simulink model "part1"  (R2025a)
settings: Solver=FixedStepAuto  StartTime=0.0  StopTime=t_end  FixedStep=dt  RelTol=1e-3
values from neighbouring files (symbols this model uses):
  alpha = wind_coeff(:,1)*pi/180    [windCoefficients.m]
  C_pitch = wind_coeff(:,6)    [windCoefficients.m]
  C_roll = wind_coeff(:,5)    [windCoefficients.m]
  C_yaw = wind_coeff(:,7)    [windCoefficients.m]
  Cx = wind_coeff(:,2)    [windCoefficients.m]
  Cy = wind_coeff(:,3)    [windCoefficients.m]
  Cz = wind_coeff(:,4)    [windCoefficients.m]
  Kd = diag([9.3e5 7e5 4e6])    [init.m]
  Ki = diag([8.5e3 7.5e3 3.5e4])    [init.m]
  Kp = diag([7.8e5   9.8e5   1.5e8])    [init.m]    (also in init_pid.m = M*Omega_n^2)
  mu = 0.001    [SimulationParam.m]
  U_bar = 10    [SimulationParam.m]
  Vc = -0.2    [SimulationParam.m]
  vessel = computeManeuveringModel(vessel, omega_p, plotFlag)    [init_pid.m]
undefined symbols (not defined in the file or in its folder): currentMode, DiscIntNeverNeededParam, Hoerner, thrusters, windFlag
libraries: marine_gnc x1, marine_hydro x1, simulink x1
settings Model: Creator=jonbjor  LastModifiedBy=evenf
settings SolverCC: AlgebraicLoopSolver=TrustRegion
settings DataIOCC: ReturnWorkspaceOutputs=off
settings DebuggingCC: UnconnectedInputMsg=warning  UnconnectedOutputMsg=warning  UnconnectedLineMsg=warning  ArithmeticOperatorsInVariantConditions=warning
settings ModelReferenceCC: EnableRefExpFcnMdlSchedulingChecks=on
settings SFSimCC: SimUseLocalCustomCode=off  CustomCodeUndefinedFunction=UseInterfaceOnly
settings RTWCC: RTWUseLocalCustomCode=off  GPUComputeCapability=3.5  DLArmComputeVersion=19.05

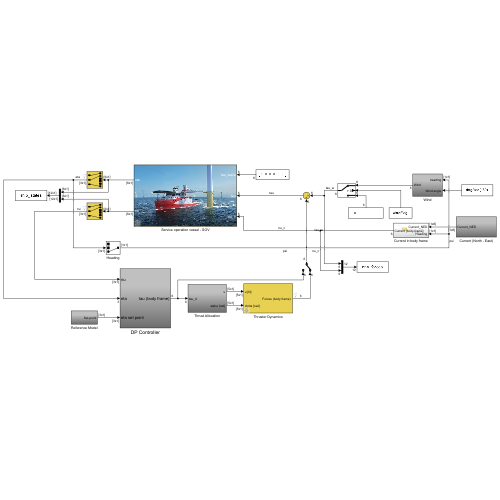
[thumbnail: Simulink's stored preview of the top-level diagram]
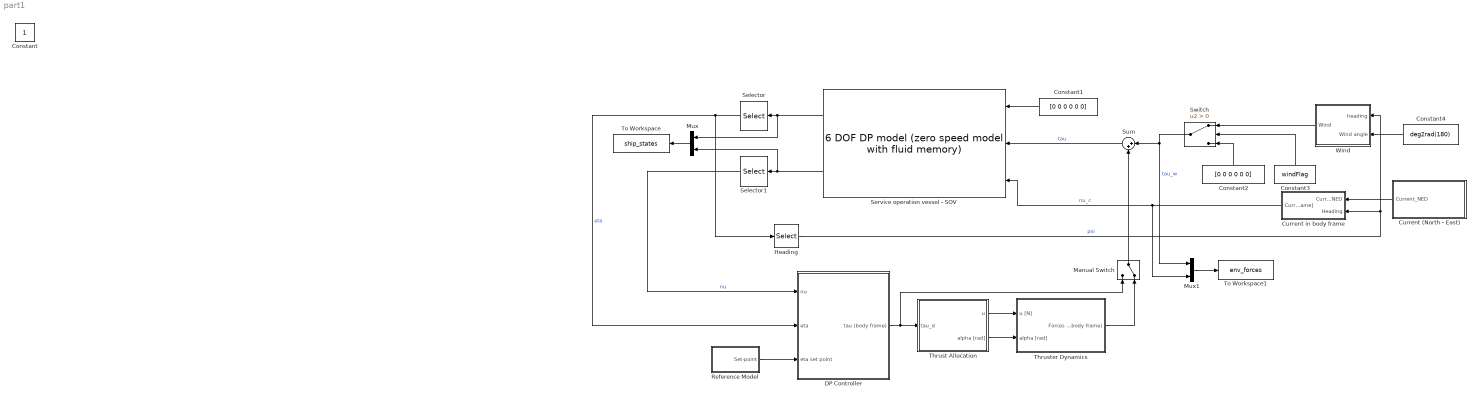
== system part1 ==
  Constant1 : Constant  Value=[0 0 0 0 0 0]
  Constant2 : Constant  Value=[0 0 0 0 0 0]
  Constant3 : Constant  Value=windFlag
  Constant4 : Constant  Value=deg2rad(180)
  Current (North - East) : Subsystem
  Current in body frame : Subsystem
  DP Controller : Subsystem
  Heading : Selector  InputPortWidth=3  IndexOptions=Index vector (dialog)  Indices=[3]  OutputSizes=1
  Manual Switch : ManualSwitch  CurrentSetting=0
  Mux : Mux  Inputs=2
  Mux1 : Mux  Inputs=2
  Reference Model : Subsystem
  Selector : Selector  InputPortWidth=6  IndexOptions=Index vector (dialog)  Indices=[1 2 6]  OutputSizes=1
  Selector1 : Selector  InputPortWidth=6  IndexOptions=Index vector (dialog)  Indices=[1 2 6]  OutputSizes=1
  Service operation vessel - SOV : marine_hydro/Hydro Library/6 DOF DP model  (zero speed model with fluid memory)  ABC=vesselABC  rho=1025  Axc=0.9*vessel.main.T*vessel.main.B  Ayc=0.9*vessel.main.T*vessel.main.Lpp  CX=1  CY_2D=Hoerner(vessel.main.B,vessel.main.T)  Bv=vessel.Bv  mask(6 DOF zero speed model){}
      link override "Integrator1 ": InitialCondition=nu0
      link override Integrator2: InitialCondition=eta0
      settings: SourceProductName=MSS Hydro
      mask Display:
      | image('SOV.jpg');
      | color('white'); port_label('output', 1, 'eta')
      | color('white'); port_label('output', 2, 'nu')
      | color('white'); port_label('input', 1, 'tau_wave')
      | color('white'); port_label('input', 2, 'tau')
      | color('white'); port_label('input', 3, 'nu_c')
  Sum : Sum  Inputs=|++
  Switch : Switch  Criteria=u2 > Threshold  SaturateOnIntegerOverflow=off  InputSameDT=off
  Thrust Allocation : Subsystem
  Thruster Dynamics : Subsystem  mask{thrusterfault=off}
      mask prompts: thrusterfault "Fault on thruster #2 and #4?"
  To Workspace : ToWorkspace  VariableName=ship_states  SampleTime=-1
  To Workspace1 : ToWorkspace  VariableName=env_forces  SampleTime=-1
      settings: Save2DSignal=2-D array (concatenate along first dimension)
  Wind : Subsystem
  Constant : Constant  IOType=siggen
  wires:
  Service operation vessel - SOV/1 -> Mux/1, Selector/1
  Service operation vessel - SOV/2 -> Mux/2, Selector1/1
  Selector/1 -> Heading/1, DP Controller/2(eta)  "eta"
  Selector1/1 -> DP Controller/1(nu)  "nu"
  Thrust Allocation/1(u) -> Thruster Dynamics/1(u [N])
  Thrust Allocation/2(alpha [rad]) -> Thruster Dynamics/2(alpha [rad])
  DP Controller/1(tau (body frame)) -> Thrust Allocation/1(tau_d), Manual Switch/1
  Sum/1 -> Service operation vessel - SOV/2  "tau"
  Current (North - East)/1(Current_NED) -> Current in body frame/1(Current_NED)
  Heading/1 -> Current in body frame/2(Heading), Wind/1(heading)  "psi"
  Current in body frame/1(Current [body-frame]) -> Service operation vessel - SOV/3, Mux1/2  "nu_c"
  Switch/1 -> Sum/1, Mux1/1  "tau_w"
  Manual Switch/1 -> Sum/2
  Thruster Dynamics/1("Forces (body frame) ") -> Manual Switch/2
  Reference Model/1(Set-point) -> DP Controller/3(eta set point)
  Mux/1 -> To Workspace/1
  Mux1/1 -> To Workspace1/1
  Constant3/1 -> Switch/2
  Constant2/1 -> Switch/3
  Wind/1(Wind) -> Switch/1
  Constant1/1 -> Service operation vessel - SOV/1
  Constant4/1 -> Wind/2(Wind angle)

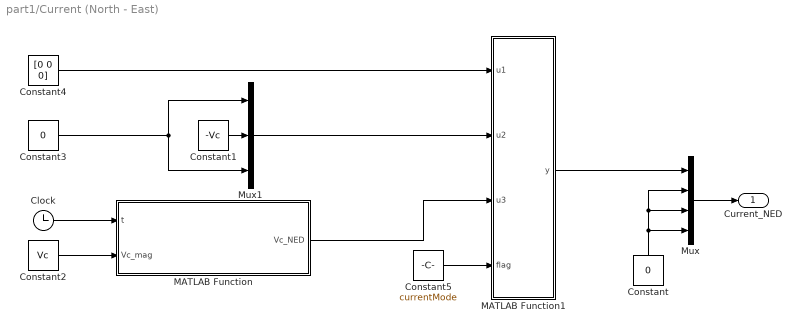
== system part1/Current (North - East) ==
  Clock : Clock
  Constant : Constant  Value=0
  Constant1 : Constant  Value=-Vc
  Constant2 : Constant  Value=Vc
  Constant3 : Constant  Value=0
  Constant4 : Constant  Value=[0 0 0]
  Constant5 : Constant  Value=currentMode
  MATLAB Function : MATLAB Function  TreatAsAtomicUnit=on
  MATLAB Function1 : MATLAB Function  TreatAsAtomicUnit=on
  Mux : Mux
  Mux1 : Mux  Inputs=3
  Current_NED : Outport  VectorParamsAs1DForOutWhenUnconnected=off
  wires:
  Constant1/1 -> Mux1/2
  Constant3/1 -> Mux1/1, Mux1/3
  Clock/1 -> MATLAB Function/1(t)
  Constant2/1 -> MATLAB Function/2(Vc_mag)
  Mux/1 -> Current_NED/1
  Constant/1 -> Mux/2, Mux/3, Mux/4
  Mux1/1 -> MATLAB Function1/2(u2)
  MATLAB Function/1(Vc_NED) -> MATLAB Function1/3(u3)
  Constant4/1 -> MATLAB Function1/1(u1)
  Constant5/1 -> MATLAB Function1/4(flag)
  MATLAB Function1/1(y) -> Mux/1

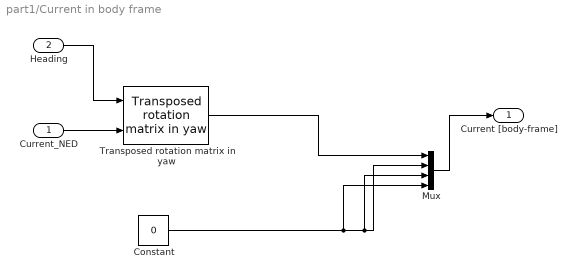
== system part1/Current in body frame ==
  Current_NED : Inport
  Heading : Inport  Port=2
  Constant : Constant  Value=0
  Mux : Mux
  Transposed rotation matrix in yaw : marine_gnc/Models/ Kinematics/Transposed rotation  matrix in yaw
      settings: SourceProductName=MSS GNC
  Current [body-frame] : Outport
  wires:
  Current_NED/1 -> Transposed rotation matrix in yaw/2
  Transposed rotation matrix in yaw/1 -> Mux/1
  Heading/1 -> Transposed rotation matrix in yaw/1
  Mux/1 -> Current [body-frame]/1
  Constant/1 -> Mux/4, Mux/3, Mux/2

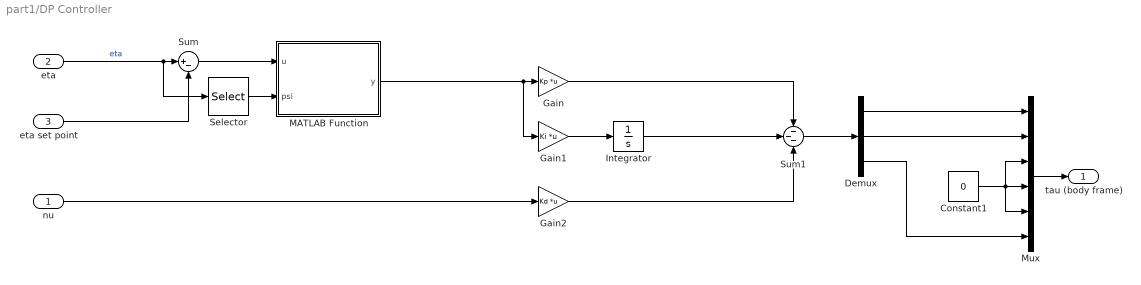
== system part1/DP Controller ==
  nu : Inport
  eta : Inport  Port=2
  eta set point : Inport  Port=3
  Constant1 : Constant  Value=0
  Demux : Demux  Outputs=3
  Gain : Gain  Gain=Kp  Multiplication=Matrix(K*u)
  Gain1 : Gain  Gain=Ki  Multiplication=Matrix(K*u)
  Gain2 : Gain  Gain=Kd  Multiplication=Matrix(K*u)
  Integrator : Integrator
  MATLAB Function : MATLAB Function  TreatAsAtomicUnit=on
  Mux : Mux  Inputs=6
  Selector : Selector  InputPortWidth=3  IndexOptions=Index vector (dialog)  Indices=[3]  OutputSizes=1
  Sum : Sum  Inputs=|+-
  Sum1 : Sum  Inputs=---
  tau (body frame) : Outport  VectorParamsAs1DForOutWhenUnconnected=off
  wires:
  Mux/1 -> tau (body frame)/1
  Constant1/1 -> Mux/5, Mux/3, Mux/4
  eta/1 -> Selector/1, Sum/1  "eta"
  eta set point/1 -> Sum/2
  Selector/1 -> MATLAB Function/2(psi)
  Sum/1 -> MATLAB Function/1(u)
  MATLAB Function/1(y) -> Gain1/1, Gain/1
  Gain1/1 -> Integrator/1
  Integrator/1 -> Sum1/2
  Gain/1 -> Sum1/1
  Sum1/1 -> Demux/1
  Demux/1 -> Mux/1
  Demux/3 -> Mux/6
  Demux/2 -> Mux/2
  nu/1 -> Gain2/1
  Gain2/1 -> Sum1/3

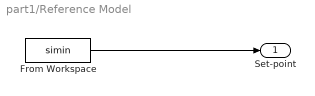
== system part1/Reference Model ==
  From Workspace : FromWorkspace  VariableName=simin
  Set-point : Outport  VectorParamsAs1DForOutWhenUnconnected=off
  wires:
  From Workspace/1 -> Set-point/1

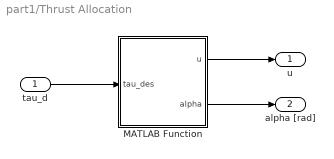
== system part1/Thrust Allocation ==
  tau_d : Inport
  MATLAB Function : MATLAB Function  TreatAsAtomicUnit=on
  u : Outport  VectorParamsAs1DForOutWhenUnconnected=off
  alpha [rad] : Outport  Port=2  VectorParamsAs1DForOutWhenUnconnected=off
  wires:
  MATLAB Function/1(u) -> u/1
  MATLAB Function/2(alpha) -> alpha [rad]/1
  tau_d/1 -> MATLAB Function/1(tau_des)

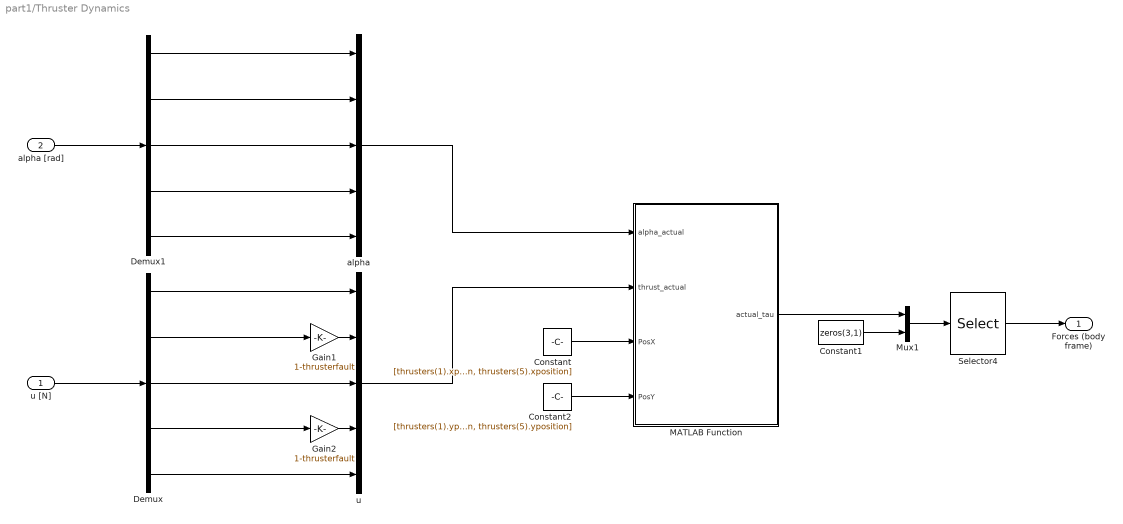
== system part1/Thruster Dynamics ==
  u [N] : Inport
  alpha [rad] : Inport  Port=2
  Constant : Constant  Value=[thrusters(1).xposition, thrusters(2).xposition, thrusters(3).xposition, thrusters(4).xposition, thrusters(5).xposition]
  Constant1 : Constant  Value=zeros(3,1)
  Constant2 : Constant  Value=[thrusters(1).yposition, thrusters(2).yposition, thrusters(3).yposition, thrusters(4).yposition, thrusters(5).yposition]
  Demux : Demux  Outputs=5
  Demux1 : Demux  Outputs=5
  Gain1 : Gain  Gain=1-thrusterfault
  Gain2 : Gain  Gain=1-thrusterfault
  MATLAB Function : MATLAB Function  TreatAsAtomicUnit=on
  Mux1 : Mux  Inputs=2
  Selector4 : Selector  InputPortWidth=6  IndexOptions=Index vector (dialog)  Indices=[1 2 4 5 6 3]  OutputSizes=1
  alpha : Mux  Inputs=5
  u : Mux  Inputs=5
  "Forces (body frame) " : Outport  VectorParamsAs1DForOutWhenUnconnected=off
  wires:
  Mux1/1 -> Selector4/1
  Constant1/1 -> Mux1/2
  Selector4/1 -> "Forces (body frame) "/1
  Gain1/1 -> u/2
  u [N]/1 -> Demux/1
  alpha [rad]/1 -> Demux1/1
  Constant/1 -> MATLAB Function/3(PosX)
  Constant2/1 -> MATLAB Function/4(PosY)
  u/1 -> MATLAB Function/2(thrust_actual)
  alpha/1 -> MATLAB Function/1(alpha_actual)
  MATLAB Function/1(actual_tau) -> Mux1/1
  Demux1/1 -> alpha/1
  Gain2/1 -> u/4
  Demux/1 -> u/1
  Demux/2 -> Gain1/1
  Demux/3 -> u/3
  Demux/4 -> Gain2/1
  Demux/5 -> u/5
  Demux1/2 -> alpha/2
  Demux1/4 -> alpha/4
  Demux1/5 -> alpha/5
  Demux1/3 -> alpha/3

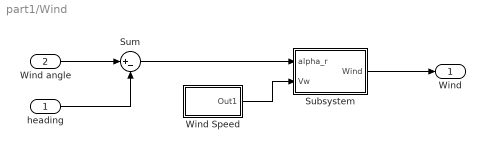
== system part1/Wind ==
  heading : Inport
  Wind angle : Inport  Port=2
  Subsystem : Subsystem
  Sum : Sum  Inputs=|+-
  Wind Speed : Subsystem
  Wind : Outport  VectorParamsAs1DForOutWhenUnconnected=off
  wires:
  Subsystem/1(Wind) -> Wind/1
  Wind Speed/1(Out1) -> Subsystem/2(Vw)
  Wind angle/1 -> Sum/1
  heading/1 -> Sum/2
  Sum/1 -> Subsystem/1(alpha_r)

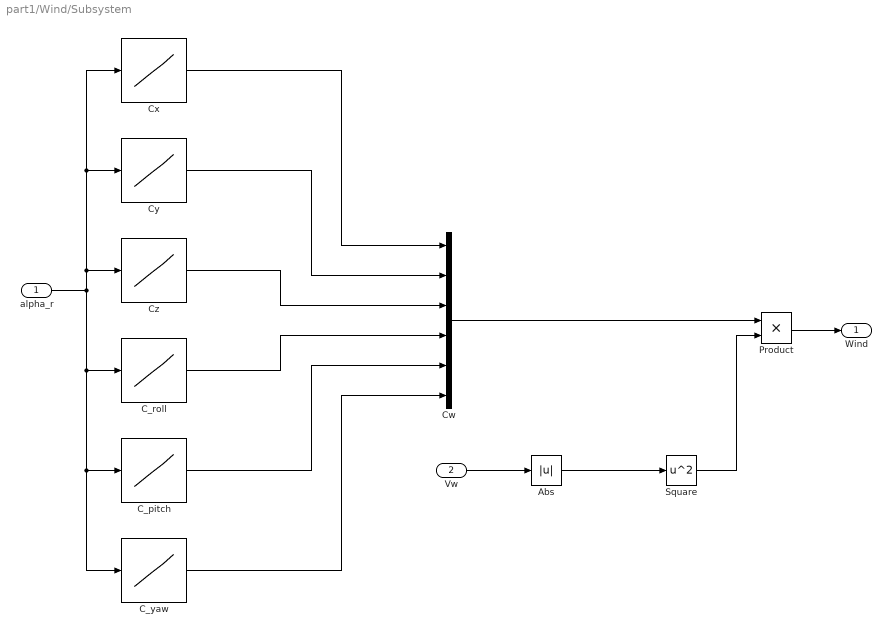
== system part1/Wind/Subsystem ==
  alpha_r : Inport
  Vw : Inport  Port=2
  Abs : Abs  SaturateOnIntegerOverflow=off
  C_pitch : Lookup_n-D  NumberOfTableDimensions=1  BreakpointsForDimension1=alpha  Table=C_pitch  InternalRulePriority=Speed  RndMeth=Simplest
  C_roll : Lookup_n-D  NumberOfTableDimensions=1  BreakpointsForDimension1=alpha  Table=C_roll  InternalRulePriority=Speed  RndMeth=Simplest
  C_yaw : Lookup_n-D  NumberOfTableDimensions=1  BreakpointsForDimension1=alpha  Table=C_yaw  InternalRulePriority=Speed  RndMeth=Simplest
  Cw : Mux  Inputs=6
  Cx : Lookup_n-D  NumberOfTableDimensions=1  BreakpointsForDimension1=alpha  Table=Cx  InternalRulePriority=Speed  RndMeth=Simplest
  Cy : Lookup_n-D  NumberOfTableDimensions=1  BreakpointsForDimension1=alpha  Table=Cy  InternalRulePriority=Speed  RndMeth=Simplest
  Cz : Lookup_n-D  NumberOfTableDimensions=1  BreakpointsForDimension1=alpha  Table=Cz  InternalRulePriority=Speed  RndMeth=Simplest
  Product : Product
  Square : Math  Operator=square
  Wind : Outport  VectorParamsAs1DForOutWhenUnconnected=off
  wires:
  Vw/1 -> Abs/1
  Cy/1 -> Cw/2
  C_roll/1 -> Cw/4
  Cw/1 -> Product/1
  C_pitch/1 -> Cw/5
  Square/1 -> Product/2
  alpha_r/1 -> C_yaw/1, C_pitch/1, C_roll/1, Cx/1, Cy/1, Cz/1
  Cz/1 -> Cw/3
  C_yaw/1 -> Cw/6
  Cx/1 -> Cw/1
  Abs/1 -> Square/1
  Product/1 -> Wind/1

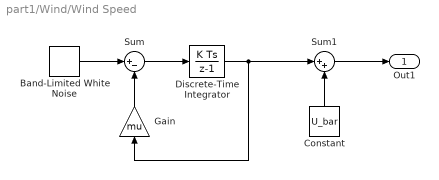
== system part1/Wind/Wind Speed ==
  Band-Limited White Noise : simulink/Sources/Band-Limited White Noise  Cov=power_w_c  Ts=0.1  seed=[23341]
  Constant : Constant  Value=U_bar
  Discrete-Time Integrator : DiscreteIntegrator  SampleTime=-1  ICPrevOutput=DiscIntNeverNeededParam  ICPrevScaledInput=DiscIntNeverNeededParam
  Gain : Gain  Gain=mu
  Sum : Sum  Inputs=|+-
  Sum1 : Sum  Inputs=|++
  Out1 : Outport
  wires:
  Discrete-Time Integrator/1 -> Gain/1, Sum1/1
  Gain/1 -> Sum/2
  Constant/1 -> Sum1/2
  Sum/1 -> Discrete-Time Integrator/1
  Band-Limited White Noise/1 -> Sum/1
  Sum1/1 -> Out1/1

== matlab function part1/Thrust Allocation/MATLAB Function ==
  data: tau_des input; u output; alpha output
function [u, alpha] = alloc_dp(tau_des)
% tau_des: desired generalized forces [X; Y; N] (3x1)
% Returns:
%   u      : [u1; u2; u3; u4; u5]
%   alpha  : [a1; a2; a3; a4; a5] 
%   Ue     : elemental vector [u1y, u2x, u2y, u3y, u4x, u4y, u5x, u5y]

% ---- geometry (body frame: +x fwd, +y stb, +N ccw)
T1 = [0; 1; 39.3];                 % tunnel bow (x=39.3, y=0)
T2 = [1 0; 0 1; 0 36.5];           % azimuth @ (x=36.5, y=0)
T3 = [0; 1; 34.4];                 % tunnel bow (x=34.4)
T4 = [1 0; 0 1; -5 -28.5];         % azimuth @ (x=-28.5, y=+5)
T5 = [1 0; 0 1;  5 -28.5];         % azimuth @ (x=-28.5, y=-5)
T  = [T1 T2 T3 T4 T5];             % 3x8: [u1y, u2x, u2y, u3y, u4x, u4y, u5x, u5y]

% ---- make sure tau is 3x1
if numel(tau_des)==6
    tau3 = [tau_des(1); tau_des(2); tau_des(6)];
else
    tau3 = tau_des(:);
end

% ---- damped least squares (better than raw pinv)
% lambda = 1e-3;                           % small Tikhonov damping
% Ue = (T.'/(T*T.' + (lambda^2)*eye(3))) * tau3;
Ue = T'*invQR( T * T')*tau3;

% ---- convert elemental components to actuator setpoints
% tunnels (signed sway)
u1 = Ue(1);           a1 =  pi/2 * sign(u1);  % sway +y is +pi/2; encode sign in angle
u3 = Ue(4);           a3 =  pi/2 * sign(u3);

% azimuth 2
Fx = Ue(2); Fy = Ue(3);
u2 = hypot(Fx,Fy);    a2 = atan2(Fy,Fx);
if u2 < 0, u2 = -u2; a2 = a2 + pi; end
a2 = wrapToPi(a2);

% azimuth 4
Fx = Ue(5); Fy = Ue(6);
u4 = hypot(Fx,Fy);    a4 = atan2(Fy,Fx);
if u4 < 0, u4 = -u4; a4 = a4 + pi; end
a4 = wrapToPi(a4);

% azimuth 5
Fx = Ue(7); Fy = Ue(8);
u5 = hypot(Fx,Fy);    a5 = atan2(Fy,Fx);
if u5 < 0, u5 = -u5; a5 = a5 + pi; end
a5 = wrapToPi(a5);

u     = [abs(u1); u2; abs(u3); u4; u5];
alpha = [a1; a2; a3; a4; a5];

end

== matlab function part1/Current (North - East)/MATLAB Function ==
  data: t input; Vc_NED output; Vc_mag input
function Vc_NED = LinearlyVaryingCurrent(t,Vc_mag)
theta = min(pi/2, (pi/2)*(t/300));  % angle in radians
Vc_NED = [Vc_mag*cos(theta) Vc_mag*sin(theta) 0];

== matlab function part1/DP Controller/MATLAB Function ==
  data: u input; y output; psi input
function y = Rz_transposed(u, psi)

y = Rzyx(0,0,psi)'*u;

== matlab function part1/Thruster Dynamics/MATLAB Function ==
  data: alpha_actual input; thrust_actual input; actual_tau output; PosX input; PosY input
function actual_tau   = fcn(alpha_actual,thrust_actual,PosX,PosY)

    Alpha_surge =[cos(alpha_actual(1)) cos(alpha_actual(2)) cos(alpha_actual(3)) cos(alpha_actual(4)) cos(alpha_actual(5))];  
    Alpha_sway = [sin(alpha_actual(1)) sin(alpha_actual(2)) sin(alpha_actual(3)) sin(alpha_actual(4)) sin(alpha_actual(5))];
    Alpha_yaw = [sin(alpha_actual(1))*PosX(1)-cos(alpha_actual(1))*PosY(1) sin(alpha_actual(2))*PosX(2)-cos(alpha_actual(2))*PosY(2) ...
                 sin(alpha_actual(3))*PosX(3)-cos(alpha_actual(3))*PosY(3) sin(alpha_actual(4))*PosX(4)-cos(alpha_actual(4))*PosY(4) ...
                 sin(alpha_actual(5))*PosX(5)-cos(alpha_actual(5))*PosY(5)];

    actual_tau = [Alpha_surge; Alpha_sway; Alpha_yaw]*thrust_actual;
end

== matlab function part1/Current (North - East)/MATLAB Function1 ==
  data: u1 input; y output; u2 input; u3 input; flag input
function y = fcn(u1, u2, u3, flag)

y = zeros(1,3);
switch flag
    case 1
        y(1:3) = u1;
    case 2
        y(1:3) = u2;
    case 3
        y(1:3) = u3;
    otherwise
        y(1:3) = u1;
end
